simulink model "TST_InjCrv_PiIAddCor"  (R2016b)
settings: Solver=FixedStepDiscrete  StartTime=0.0  StopTime=simTime  FixedStep=sampleTime  RelTol=1e-3
values from neighbouring files (symbols this model uses):
  testCase = 1    [initTST_InjCrv_PiIAddCor_001.m]    (also in initTST_InjCrv_PiIAddCor_002.m = 2; initTST_InjCrv_PiIAddCor_003.m = 3)
libraries: simulink x7
settings Model: Creator=WF305  LastModifiedBy=WF305
settings DebuggingCC: SignalRangeChecking=error

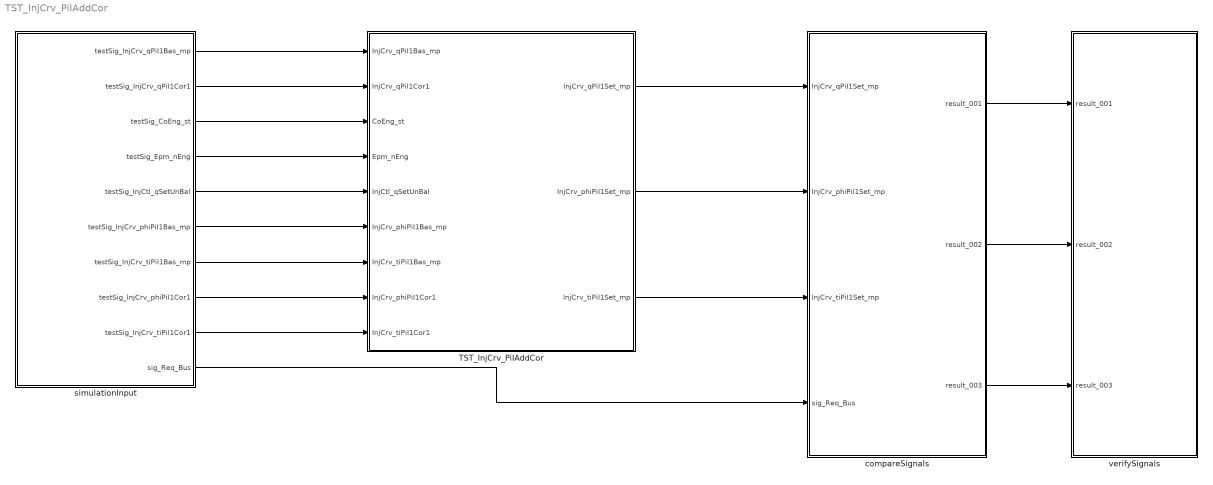
== system TST_InjCrv_PiIAddCor ==
  TST_InjCrv_PiIAddCor : Subsystem
  compareSignals : Subsystem
  simulationInput : Subsystem
  verifySignals : Subsystem
  wires:
  simulationInput/1(testSig_InjCrv_qPiI1Bas_mp) -> TST_InjCrv_PiIAddCor/1(InjCrv_qPiI1Bas_mp)
  simulationInput/2(testSig_InjCrv_qPiI1Cor1) -> TST_InjCrv_PiIAddCor/2(InjCrv_qPiI1Cor1)
  simulationInput/3(testSig_CoEng_st) -> TST_InjCrv_PiIAddCor/3(CoEng_st)
  simulationInput/4(testSig_Epm_nEng) -> TST_InjCrv_PiIAddCor/4(Epm_nEng)
  simulationInput/5(testSig_InjCtl_qSetUnBal) -> TST_InjCrv_PiIAddCor/5(InjCtl_qSetUnBal)
  simulationInput/6(testSig_InjCrv_phiPiI1Bas_mp) -> TST_InjCrv_PiIAddCor/6(InjCrv_phiPiI1Bas_mp)
  simulationInput/7(testSig_InjCrv_tiPiI1Bas_mp) -> TST_InjCrv_PiIAddCor/7(InjCrv_tiPiI1Bas_mp)
  simulationInput/8(testSig_InjCrv_phiPiI1Cor1) -> TST_InjCrv_PiIAddCor/8(InjCrv_phiPiI1Cor1)
  simulationInput/9(testSig_InjCrv_tiPiI1Cor1) -> TST_InjCrv_PiIAddCor/9(InjCrv_tiPiI1Cor1)
  TST_InjCrv_PiIAddCor/1(InjCrv_qPiI1Set_mp) -> compareSignals/1(InjCrv_qPiI1Set_mp)
  TST_InjCrv_PiIAddCor/2(InjCrv_phiPiI1Set_mp) -> compareSignals/2(InjCrv_phiPiI1Set_mp)
  TST_InjCrv_PiIAddCor/3(InjCrv_tiPiI1Set_mp) -> compareSignals/3(InjCrv_tiPiI1Set_mp)
  simulationInput/10(sig_Req_Bus) -> compareSignals/4(sig_Req_Bus)
  compareSignals/1(result_001) -> verifySignals/1(result_001)
  compareSignals/2(result_002) -> verifySignals/2(result_002)
  compareSignals/3(result_003) -> verifySignals/3(result_003)

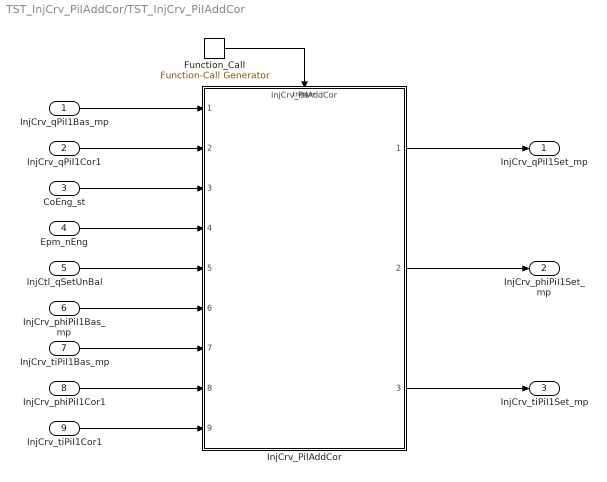
== system TST_InjCrv_PiIAddCor/TST_InjCrv_PiIAddCor ==
  InjCrv_qPiI1Bas_mp : Inport
  InjCrv_qPiI1Cor1 : Inport  Port=2
  CoEng_st : Inport  Port=3
  Epm_nEng : Inport  Port=4
  InjCtl_qSetUnBal : Inport  Port=5
  InjCrv_phiPiI1Bas_mp : Inport  Port=6
  InjCrv_tiPiI1Bas_mp : Inport  Port=7
  InjCrv_phiPiI1Cor1 : Inport  Port=8
  InjCrv_tiPiI1Cor1 : Inport  Port=9
  Function_Call : simulink/Ports & Subsystems/Function-Call Generator  sample_time=sampleTime  numberOfIterations=1
  InjCrv_PiIAddCor : ModelReference  ModelNameDialog=InjCrv_PiIAddCor  ModelReferenceVersion=1.17  TriggerPortName=function  TriggerPortTriggerType=function-call  TriggerPortStatesWhenEnabling=held
  InjCrv_qPiI1Set_mp : Outport
  InjCrv_phiPiI1Set_mp : Outport  Port=2
  InjCrv_tiPiI1Set_mp : Outport  Port=3
  wires:
  Function_Call/1 -> InjCrv_PiIAddCor/Trigger
  InjCrv_qPiI1Bas_mp/1 -> InjCrv_PiIAddCor/1
  InjCrv_qPiI1Cor1/1 -> InjCrv_PiIAddCor/2
  CoEng_st/1 -> InjCrv_PiIAddCor/3
  Epm_nEng/1 -> InjCrv_PiIAddCor/4
  InjCtl_qSetUnBal/1 -> InjCrv_PiIAddCor/5
  InjCrv_phiPiI1Bas_mp/1 -> InjCrv_PiIAddCor/6
  InjCrv_tiPiI1Bas_mp/1 -> InjCrv_PiIAddCor/7
  InjCrv_phiPiI1Cor1/1 -> InjCrv_PiIAddCor/8
  InjCrv_tiPiI1Cor1/1 -> InjCrv_PiIAddCor/9
  InjCrv_PiIAddCor/1 -> InjCrv_qPiI1Set_mp/1
  InjCrv_PiIAddCor/2 -> InjCrv_phiPiI1Set_mp/1
  InjCrv_PiIAddCor/3 -> InjCrv_tiPiI1Set_mp/1

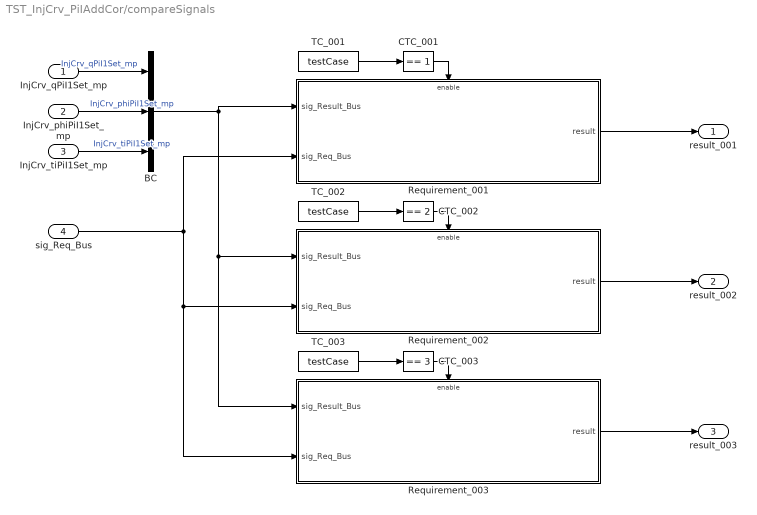
== system TST_InjCrv_PiIAddCor/compareSignals ==
  InjCrv_qPiI1Set_mp : Inport
  InjCrv_phiPiI1Set_mp : Inport  Port=2
  InjCrv_tiPiI1Set_mp : Inport  Port=3
  sig_Req_Bus : Inport  Port=4
  BC : BusCreator  Inputs=3
  CTC_001 : simulink/Logic and Bit Operations/Compare To Constant  relop===  const=1  OutDataTypeStr=boolean
  CTC_002 : simulink/Logic and Bit Operations/Compare To Constant  relop===  const=2  OutDataTypeStr=boolean
  CTC_003 : simulink/Logic and Bit Operations/Compare To Constant  relop===  const=3  OutDataTypeStr=boolean
  Requirement_001 : Subsystem
  Requirement_002 : Subsystem
  Requirement_003 : Subsystem
  TC_001 : Constant  Value=testCase
  TC_002 : Constant  Value=testCase
  TC_003 : Constant  Value=testCase
  result_001 : Outport
  result_002 : Outport  Port=2
  result_003 : Outport  Port=3
  wires:
  InjCrv_qPiI1Set_mp/1 -> BC/1  "InjCrv_qPiI1Set_mp"
  InjCrv_phiPiI1Set_mp/1 -> BC/2  "InjCrv_phiPiI1Set_mp"
  InjCrv_tiPiI1Set_mp/1 -> BC/3  "InjCrv_tiPiI1Set_mp"
  TC_001/1 -> CTC_001/1
  CTC_001/1 -> Requirement_001/Enable
  sig_Req_Bus/1 -> Requirement_002/2(sig_Req_Bus), Requirement_003/2(sig_Req_Bus), Requirement_001/2(sig_Req_Bus)
  BC/1 -> Requirement_002/1(sig_Result_Bus), Requirement_003/1(sig_Result_Bus), Requirement_001/1(sig_Result_Bus)
  Requirement_001/1(result) -> result_001/1
  TC_002/1 -> CTC_002/1
  CTC_002/1 -> Requirement_002/Enable
  Requirement_002/1(result) -> result_002/1
  TC_003/1 -> CTC_003/1
  CTC_003/1 -> Requirement_003/Enable
  Requirement_003/1(result) -> result_003/1

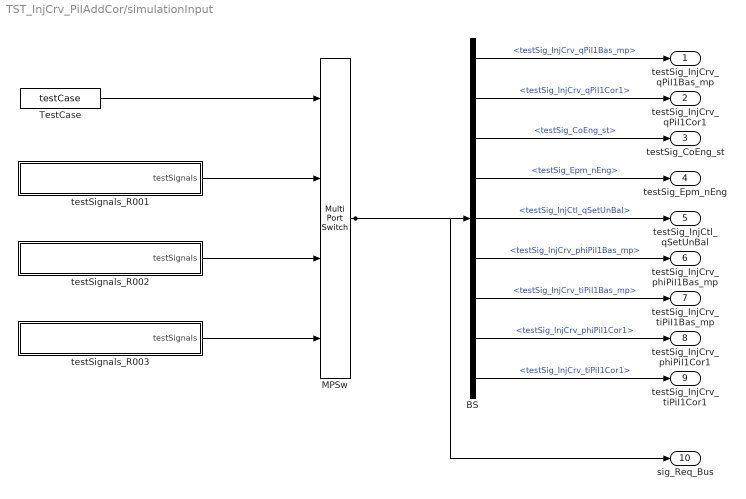
== system TST_InjCrv_PiIAddCor/simulationInput ==
  BS : BusSelector  OutputSignals=testSig_InjCrv_qPiI1Bas_mp,testSig_InjCrv_qPiI1Cor1,testSig_CoEng_st,testSig_Epm_nEng,testSig_InjCtl_qSetUnBal,testSig_InjCrv_phiPiI1Bas_mp,testSig_InjCrv_tiPiI1Bas_mp,testSig_InjCrv_phiPiI1Cor1,testSig_InjCrv_tiPiI1Cor1
  MPSw : MultiPortSwitch  SaturateOnIntegerOverflow=on  InputSameDT=on
  TestCase : Constant  Value=testCase
  testSignals_R001 : Subsystem
  testSignals_R002 : Subsystem
  testSignals_R003 : Subsystem
  testSig_InjCrv_qPiI1Bas_mp : Outport
  testSig_InjCrv_qPiI1Cor1 : Outport  Port=2
  testSig_CoEng_st : Outport  Port=3
  testSig_Epm_nEng : Outport  Port=4
  testSig_InjCtl_qSetUnBal : Outport  Port=5
  testSig_InjCrv_phiPiI1Bas_mp : Outport  Port=6
  testSig_InjCrv_tiPiI1Bas_mp : Outport  Port=7
  testSig_InjCrv_phiPiI1Cor1 : Outport  Port=8
  testSig_InjCrv_tiPiI1Cor1 : Outport  Port=9
  sig_Req_Bus : Outport  Port=10
  wires:
  BS/1 -> testSig_InjCrv_qPiI1Bas_mp/1  "<testSig_InjCrv_qPiI1Bas_mp>"
  BS/2 -> testSig_InjCrv_qPiI1Cor1/1  "<testSig_InjCrv_qPiI1Cor1>"
  BS/3 -> testSig_CoEng_st/1  "<testSig_CoEng_st>"
  BS/4 -> testSig_Epm_nEng/1  "<testSig_Epm_nEng>"
  BS/5 -> testSig_InjCtl_qSetUnBal/1  "<testSig_InjCtl_qSetUnBal>"
  BS/6 -> testSig_InjCrv_phiPiI1Bas_mp/1  "<testSig_InjCrv_phiPiI1Bas_mp>"
  BS/7 -> testSig_InjCrv_tiPiI1Bas_mp/1  "<testSig_InjCrv_tiPiI1Bas_mp>"
  BS/8 -> testSig_InjCrv_phiPiI1Cor1/1  "<testSig_InjCrv_phiPiI1Cor1>"
  BS/9 -> testSig_InjCrv_tiPiI1Cor1/1  "<testSig_InjCrv_tiPiI1Cor1>"
  MPSw/1 -> BS/1, sig_Req_Bus/1
  TestCase/1 -> MPSw/1
  testSignals_R001/1(testSignals) -> MPSw/2
  testSignals_R002/1(testSignals) -> MPSw/3
  testSignals_R003/1(testSignals) -> MPSw/4

== system TST_InjCrv_PiIAddCor/verifySignals ==
  result_001 : Inport
  result_002 : Inport  Port=2
  result_003 : Inport  Port=3
  Assertion_001 : Assertion  Enabled=off
  Assertion_002 : Assertion  Enabled=off
  Assertion_003 : Assertion  Enabled=off
  wires:
  result_001/1 -> Assertion_001/1
  result_002/1 -> Assertion_002/1
  result_003/1 -> Assertion_003/1

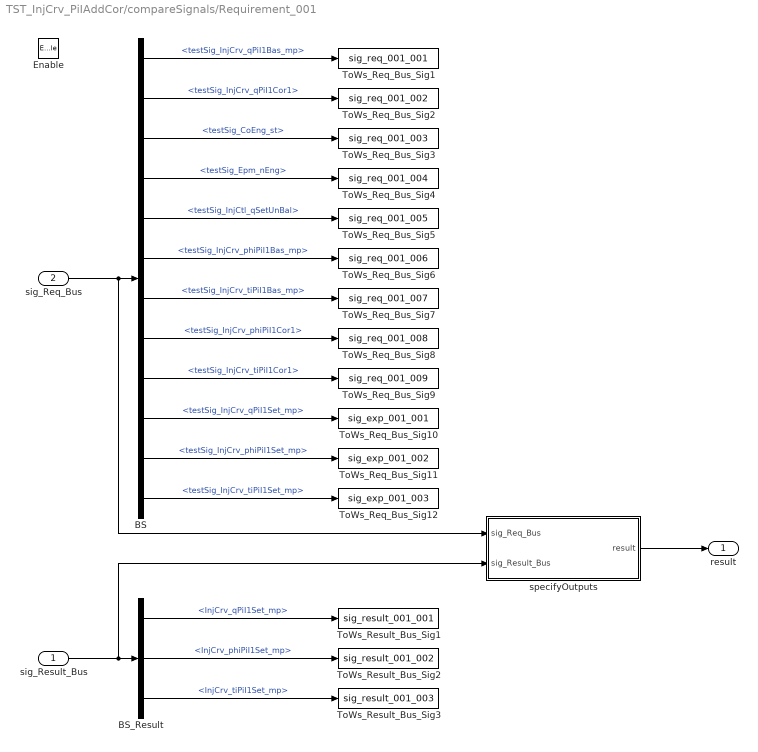
== system TST_InjCrv_PiIAddCor/compareSignals/Requirement_001 ==
  sig_Result_Bus : Inport
  sig_Req_Bus : Inport  Port=2
  Enable : EnablePort
  BS : BusSelector  OutputSignals=testSig_InjCrv_qPiI1Bas_mp,testSig_InjCrv_qPiI1Cor1,testSig_CoEng_st,testSig_Epm_nEng,testSig_InjCtl_qSetUnBal,testSig_InjCrv_phiPiI1Bas_mp,testSig_InjCrv_tiPiI1Bas_mp,testSig_InjCrv_phiPiI1Cor1,testSig_InjCrv_tiPiI1Cor1,testSig_InjCrv_qPiI1Set_mp,testSig_InjCrv_phiPiI1Set_mp,testSig_InjCrv_tiPiI1Set_mp
  BS_Result : BusSelector  OutputSignals=InjCrv_qPiI1Set_mp,InjCrv_phiPiI1Set_mp,InjCrv_tiPiI1Set_mp
  ToWs_Req_Bus_Sig1 : ToWorkspace  VariableName=sig_req_001_001  SaveFormat=Structure With Time
  ToWs_Req_Bus_Sig10 : ToWorkspace  VariableName=sig_exp_001_001  SaveFormat=Structure With Time
  ToWs_Req_Bus_Sig11 : ToWorkspace  VariableName=sig_exp_001_002  SaveFormat=Structure With Time
  ToWs_Req_Bus_Sig12 : ToWorkspace  VariableName=sig_exp_001_003  SaveFormat=Structure With Time
  ToWs_Req_Bus_Sig2 : ToWorkspace  VariableName=sig_req_001_002  SaveFormat=Structure With Time
  ToWs_Req_Bus_Sig3 : ToWorkspace  VariableName=sig_req_001_003  SaveFormat=Structure With Time
  ToWs_Req_Bus_Sig4 : ToWorkspace  VariableName=sig_req_001_004  SaveFormat=Structure With Time
  ToWs_Req_Bus_Sig5 : ToWorkspace  VariableName=sig_req_001_005  SaveFormat=Structure With Time
  ToWs_Req_Bus_Sig6 : ToWorkspace  VariableName=sig_req_001_006  SaveFormat=Structure With Time
  ToWs_Req_Bus_Sig7 : ToWorkspace  VariableName=sig_req_001_007  SaveFormat=Structure With Time
  ToWs_Req_Bus_Sig8 : ToWorkspace  VariableName=sig_req_001_008  SaveFormat=Structure With Time
  ToWs_Req_Bus_Sig9 : ToWorkspace  VariableName=sig_req_001_009  SaveFormat=Structure With Time
  ToWs_Result_Bus_Sig1 : ToWorkspace  VariableName=sig_result_001_001  SaveFormat=Structure With Time
  ToWs_Result_Bus_Sig2 : ToWorkspace  VariableName=sig_result_001_002  SaveFormat=Structure With Time
  ToWs_Result_Bus_Sig3 : ToWorkspace  VariableName=sig_result_001_003  SaveFormat=Structure With Time
  specifyOutputs : Subsystem
  result : Outport
  wires:
  sig_Req_Bus/1 -> BS/1, specifyOutputs/1(sig_Req_Bus)
  BS/1 -> ToWs_Req_Bus_Sig1/1  "<testSig_InjCrv_qPiI1Bas_mp>"
  BS/2 -> ToWs_Req_Bus_Sig2/1  "<testSig_InjCrv_qPiI1Cor1>"
  BS/3 -> ToWs_Req_Bus_Sig3/1  "<testSig_CoEng_st>"
  BS/4 -> ToWs_Req_Bus_Sig4/1  "<testSig_Epm_nEng>"
  BS/5 -> ToWs_Req_Bus_Sig5/1  "<testSig_InjCtl_qSetUnBal>"
  BS/6 -> ToWs_Req_Bus_Sig6/1  "<testSig_InjCrv_phiPiI1Bas_mp>"
  BS/7 -> ToWs_Req_Bus_Sig7/1  "<testSig_InjCrv_tiPiI1Bas_mp>"
  BS/8 -> ToWs_Req_Bus_Sig8/1  "<testSig_InjCrv_phiPiI1Cor1>"
  BS/9 -> ToWs_Req_Bus_Sig9/1  "<testSig_InjCrv_tiPiI1Cor1>"
  BS/10 -> ToWs_Req_Bus_Sig10/1  "<testSig_InjCrv_qPiI1Set_mp>"
  BS/11 -> ToWs_Req_Bus_Sig11/1  "<testSig_InjCrv_phiPiI1Set_mp>"
  BS/12 -> ToWs_Req_Bus_Sig12/1  "<testSig_InjCrv_tiPiI1Set_mp>"
  sig_Result_Bus/1 -> BS_Result/1, specifyOutputs/2(sig_Result_Bus)
  BS_Result/1 -> ToWs_Result_Bus_Sig1/1  "<InjCrv_qPiI1Set_mp>"
  BS_Result/2 -> ToWs_Result_Bus_Sig2/1  "<InjCrv_phiPiI1Set_mp>"
  BS_Result/3 -> ToWs_Result_Bus_Sig3/1  "<InjCrv_tiPiI1Set_mp>"
  specifyOutputs/1(result) -> result/1

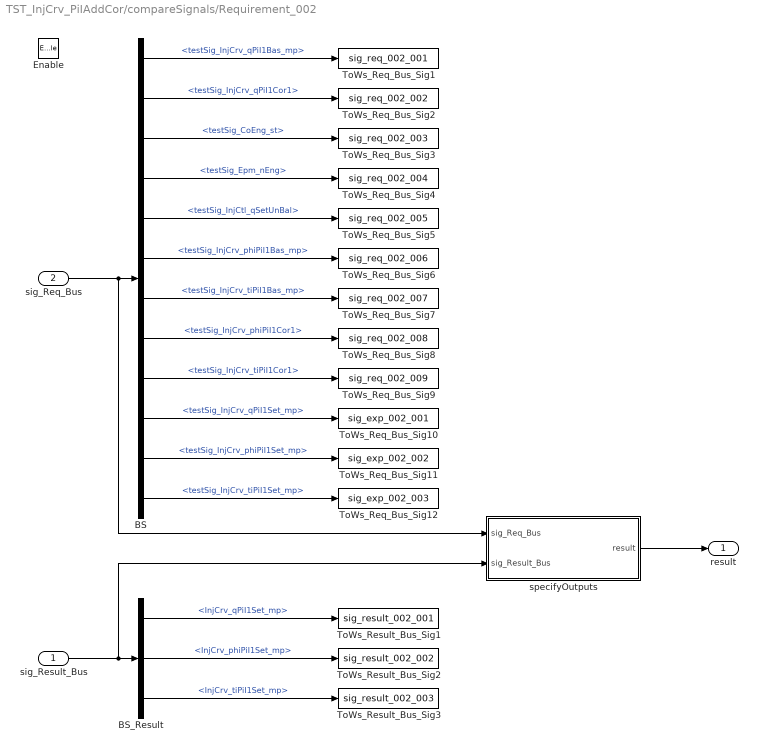
== system TST_InjCrv_PiIAddCor/compareSignals/Requirement_002 ==
  sig_Result_Bus : Inport
  sig_Req_Bus : Inport  Port=2
  Enable : EnablePort
  BS : BusSelector  OutputSignals=testSig_InjCrv_qPiI1Bas_mp,testSig_InjCrv_qPiI1Cor1,testSig_CoEng_st,testSig_Epm_nEng,testSig_InjCtl_qSetUnBal,testSig_InjCrv_phiPiI1Bas_mp,testSig_InjCrv_tiPiI1Bas_mp,testSig_InjCrv_phiPiI1Cor1,testSig_InjCrv_tiPiI1Cor1,testSig_InjCrv_qPiI1Set_mp,testSig_InjCrv_phiPiI1Set_mp,testSig_InjCrv_tiPiI1Set_mp
  BS_Result : BusSelector  OutputSignals=InjCrv_qPiI1Set_mp,InjCrv_phiPiI1Set_mp,InjCrv_tiPiI1Set_mp
  ToWs_Req_Bus_Sig1 : ToWorkspace  VariableName=sig_req_002_001  SaveFormat=Structure With Time
  ToWs_Req_Bus_Sig10 : ToWorkspace  VariableName=sig_exp_002_001  SaveFormat=Structure With Time
  ToWs_Req_Bus_Sig11 : ToWorkspace  VariableName=sig_exp_002_002  SaveFormat=Structure With Time
  ToWs_Req_Bus_Sig12 : ToWorkspace  VariableName=sig_exp_002_003  SaveFormat=Structure With Time
  ToWs_Req_Bus_Sig2 : ToWorkspace  VariableName=sig_req_002_002  SaveFormat=Structure With Time
  ToWs_Req_Bus_Sig3 : ToWorkspace  VariableName=sig_req_002_003  SaveFormat=Structure With Time
  ToWs_Req_Bus_Sig4 : ToWorkspace  VariableName=sig_req_002_004  SaveFormat=Structure With Time
  ToWs_Req_Bus_Sig5 : ToWorkspace  VariableName=sig_req_002_005  SaveFormat=Structure With Time
  ToWs_Req_Bus_Sig6 : ToWorkspace  VariableName=sig_req_002_006  SaveFormat=Structure With Time
  ToWs_Req_Bus_Sig7 : ToWorkspace  VariableName=sig_req_002_007  SaveFormat=Structure With Time
  ToWs_Req_Bus_Sig8 : ToWorkspace  VariableName=sig_req_002_008  SaveFormat=Structure With Time
  ToWs_Req_Bus_Sig9 : ToWorkspace  VariableName=sig_req_002_009  SaveFormat=Structure With Time
  ToWs_Result_Bus_Sig1 : ToWorkspace  VariableName=sig_result_002_001  SaveFormat=Structure With Time
  ToWs_Result_Bus_Sig2 : ToWorkspace  VariableName=sig_result_002_002  SaveFormat=Structure With Time
  ToWs_Result_Bus_Sig3 : ToWorkspace  VariableName=sig_result_002_003  SaveFormat=Structure With Time
  specifyOutputs : Subsystem
  result : Outport
  wires:
  sig_Req_Bus/1 -> BS/1, specifyOutputs/1(sig_Req_Bus)
  BS/1 -> ToWs_Req_Bus_Sig1/1  "<testSig_InjCrv_qPiI1Bas_mp>"
  BS/2 -> ToWs_Req_Bus_Sig2/1  "<testSig_InjCrv_qPiI1Cor1>"
  BS/3 -> ToWs_Req_Bus_Sig3/1  "<testSig_CoEng_st>"
  BS/4 -> ToWs_Req_Bus_Sig4/1  "<testSig_Epm_nEng>"
  BS/5 -> ToWs_Req_Bus_Sig5/1  "<testSig_InjCtl_qSetUnBal>"
  BS/6 -> ToWs_Req_Bus_Sig6/1  "<testSig_InjCrv_phiPiI1Bas_mp>"
  BS/7 -> ToWs_Req_Bus_Sig7/1  "<testSig_InjCrv_tiPiI1Bas_mp>"
  BS/8 -> ToWs_Req_Bus_Sig8/1  "<testSig_InjCrv_phiPiI1Cor1>"
  BS/9 -> ToWs_Req_Bus_Sig9/1  "<testSig_InjCrv_tiPiI1Cor1>"
  BS/10 -> ToWs_Req_Bus_Sig10/1  "<testSig_InjCrv_qPiI1Set_mp>"
  BS/11 -> ToWs_Req_Bus_Sig11/1  "<testSig_InjCrv_phiPiI1Set_mp>"
  BS/12 -> ToWs_Req_Bus_Sig12/1  "<testSig_InjCrv_tiPiI1Set_mp>"
  sig_Result_Bus/1 -> BS_Result/1, specifyOutputs/2(sig_Result_Bus)
  BS_Result/1 -> ToWs_Result_Bus_Sig1/1  "<InjCrv_qPiI1Set_mp>"
  BS_Result/2 -> ToWs_Result_Bus_Sig2/1  "<InjCrv_phiPiI1Set_mp>"
  BS_Result/3 -> ToWs_Result_Bus_Sig3/1  "<InjCrv_tiPiI1Set_mp>"
  specifyOutputs/1(result) -> result/1

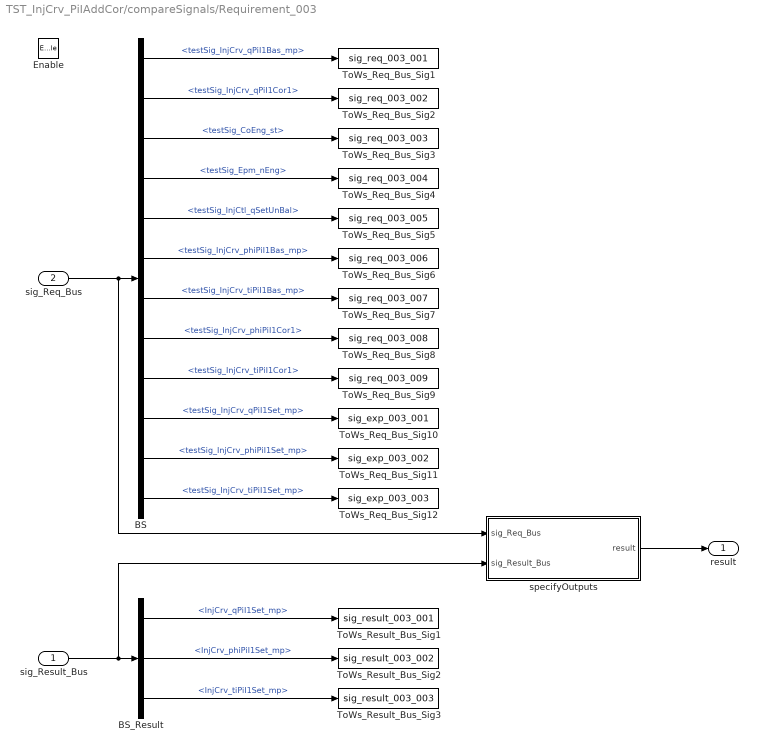
== system TST_InjCrv_PiIAddCor/compareSignals/Requirement_003 ==
  sig_Result_Bus : Inport
  sig_Req_Bus : Inport  Port=2
  Enable : EnablePort
  BS : BusSelector  OutputSignals=testSig_InjCrv_qPiI1Bas_mp,testSig_InjCrv_qPiI1Cor1,testSig_CoEng_st,testSig_Epm_nEng,testSig_InjCtl_qSetUnBal,testSig_InjCrv_phiPiI1Bas_mp,testSig_InjCrv_tiPiI1Bas_mp,testSig_InjCrv_phiPiI1Cor1,testSig_InjCrv_tiPiI1Cor1,testSig_InjCrv_qPiI1Set_mp,testSig_InjCrv_phiPiI1Set_mp,testSig_InjCrv_tiPiI1Set_mp
  BS_Result : BusSelector  OutputSignals=InjCrv_qPiI1Set_mp,InjCrv_phiPiI1Set_mp,InjCrv_tiPiI1Set_mp
  ToWs_Req_Bus_Sig1 : ToWorkspace  VariableName=sig_req_003_001  SaveFormat=Structure With Time
  ToWs_Req_Bus_Sig10 : ToWorkspace  VariableName=sig_exp_003_001  SaveFormat=Structure With Time
  ToWs_Req_Bus_Sig11 : ToWorkspace  VariableName=sig_exp_003_002  SaveFormat=Structure With Time
  ToWs_Req_Bus_Sig12 : ToWorkspace  VariableName=sig_exp_003_003  SaveFormat=Structure With Time
  ToWs_Req_Bus_Sig2 : ToWorkspace  VariableName=sig_req_003_002  SaveFormat=Structure With Time
  ToWs_Req_Bus_Sig3 : ToWorkspace  VariableName=sig_req_003_003  SaveFormat=Structure With Time
  ToWs_Req_Bus_Sig4 : ToWorkspace  VariableName=sig_req_003_004  SaveFormat=Structure With Time
  ToWs_Req_Bus_Sig5 : ToWorkspace  VariableName=sig_req_003_005  SaveFormat=Structure With Time
  ToWs_Req_Bus_Sig6 : ToWorkspace  VariableName=sig_req_003_006  SaveFormat=Structure With Time
  ToWs_Req_Bus_Sig7 : ToWorkspace  VariableName=sig_req_003_007  SaveFormat=Structure With Time
  ToWs_Req_Bus_Sig8 : ToWorkspace  VariableName=sig_req_003_008  SaveFormat=Structure With Time
  ToWs_Req_Bus_Sig9 : ToWorkspace  VariableName=sig_req_003_009  SaveFormat=Structure With Time
  ToWs_Result_Bus_Sig1 : ToWorkspace  VariableName=sig_result_003_001  SaveFormat=Structure With Time
  ToWs_Result_Bus_Sig2 : ToWorkspace  VariableName=sig_result_003_002  SaveFormat=Structure With Time
  ToWs_Result_Bus_Sig3 : ToWorkspace  VariableName=sig_result_003_003  SaveFormat=Structure With Time
  specifyOutputs : Subsystem
  result : Outport
  wires:
  sig_Req_Bus/1 -> BS/1, specifyOutputs/1(sig_Req_Bus)
  BS/1 -> ToWs_Req_Bus_Sig1/1  "<testSig_InjCrv_qPiI1Bas_mp>"
  BS/2 -> ToWs_Req_Bus_Sig2/1  "<testSig_InjCrv_qPiI1Cor1>"
  BS/3 -> ToWs_Req_Bus_Sig3/1  "<testSig_CoEng_st>"
  BS/4 -> ToWs_Req_Bus_Sig4/1  "<testSig_Epm_nEng>"
  BS/5 -> ToWs_Req_Bus_Sig5/1  "<testSig_InjCtl_qSetUnBal>"
  BS/6 -> ToWs_Req_Bus_Sig6/1  "<testSig_InjCrv_phiPiI1Bas_mp>"
  BS/7 -> ToWs_Req_Bus_Sig7/1  "<testSig_InjCrv_tiPiI1Bas_mp>"
  BS/8 -> ToWs_Req_Bus_Sig8/1  "<testSig_InjCrv_phiPiI1Cor1>"
  BS/9 -> ToWs_Req_Bus_Sig9/1  "<testSig_InjCrv_tiPiI1Cor1>"
  BS/10 -> ToWs_Req_Bus_Sig10/1  "<testSig_InjCrv_qPiI1Set_mp>"
  BS/11 -> ToWs_Req_Bus_Sig11/1  "<testSig_InjCrv_phiPiI1Set_mp>"
  BS/12 -> ToWs_Req_Bus_Sig12/1  "<testSig_InjCrv_tiPiI1Set_mp>"
  sig_Result_Bus/1 -> BS_Result/1, specifyOutputs/2(sig_Result_Bus)
  BS_Result/1 -> ToWs_Result_Bus_Sig1/1  "<InjCrv_qPiI1Set_mp>"
  BS_Result/2 -> ToWs_Result_Bus_Sig2/1  "<InjCrv_phiPiI1Set_mp>"
  BS_Result/3 -> ToWs_Result_Bus_Sig3/1  "<InjCrv_tiPiI1Set_mp>"
  specifyOutputs/1(result) -> result/1

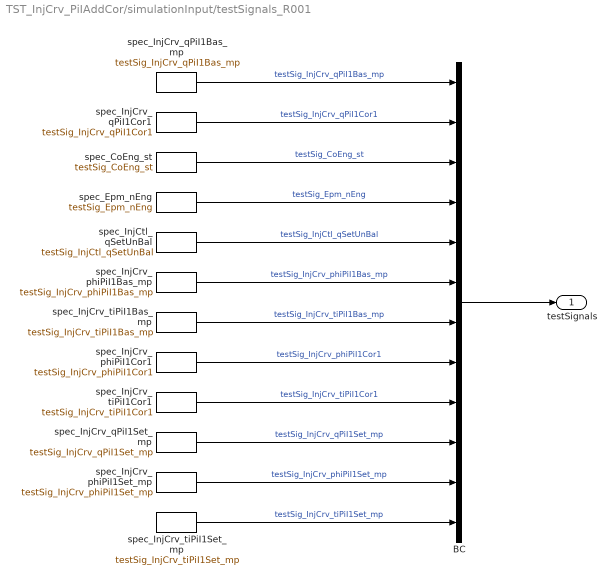
== system TST_InjCrv_PiIAddCor/simulationInput/testSignals_R001 ==
  BC : BusCreator  Inputs=12
  spec_CoEng_st : FromWorkspace  VariableName=testSig_CoEng_st  Interpolate=off  OutputAfterFinalValue=Holding final value
  spec_Epm_nEng : FromWorkspace  VariableName=testSig_Epm_nEng  Interpolate=off  OutputAfterFinalValue=Holding final value
  spec_InjCrv_phiPiI1Bas_mp : FromWorkspace  VariableName=testSig_InjCrv_phiPiI1Bas_mp  Interpolate=off  OutputAfterFinalValue=Holding final value
  spec_InjCrv_phiPiI1Cor1 : FromWorkspace  VariableName=testSig_InjCrv_phiPiI1Cor1  Interpolate=off  OutputAfterFinalValue=Holding final value
  spec_InjCrv_phiPiI1Set_mp : FromWorkspace  VariableName=testSig_InjCrv_phiPiI1Set_mp  Interpolate=off  OutputAfterFinalValue=Holding final value
  spec_InjCrv_qPiI1Bas_mp : FromWorkspace  VariableName=testSig_InjCrv_qPiI1Bas_mp  Interpolate=off  OutputAfterFinalValue=Holding final value
  spec_InjCrv_qPiI1Cor1 : FromWorkspace  VariableName=testSig_InjCrv_qPiI1Cor1  Interpolate=off  OutputAfterFinalValue=Holding final value
  spec_InjCrv_qPiI1Set_mp : FromWorkspace  VariableName=testSig_InjCrv_qPiI1Set_mp  Interpolate=off  OutputAfterFinalValue=Holding final value
  spec_InjCrv_tiPiI1Bas_mp : FromWorkspace  VariableName=testSig_InjCrv_tiPiI1Bas_mp  Interpolate=off  OutputAfterFinalValue=Holding final value
  spec_InjCrv_tiPiI1Cor1 : FromWorkspace  VariableName=testSig_InjCrv_tiPiI1Cor1  Interpolate=off  OutputAfterFinalValue=Holding final value
  spec_InjCrv_tiPiI1Set_mp : FromWorkspace  VariableName=testSig_InjCrv_tiPiI1Set_mp  Interpolate=off  OutputAfterFinalValue=Holding final value
  spec_InjCtl_qSetUnBal : FromWorkspace  VariableName=testSig_InjCtl_qSetUnBal  Interpolate=off  OutputAfterFinalValue=Holding final value
  testSignals : Outport
  wires:
  BC/1 -> testSignals/1
  spec_InjCrv_qPiI1Bas_mp/1 -> BC/1  "testSig_InjCrv_qPiI1Bas_mp"
  spec_InjCrv_qPiI1Cor1/1 -> BC/2  "testSig_InjCrv_qPiI1Cor1"
  spec_CoEng_st/1 -> BC/3  "testSig_CoEng_st"
  spec_Epm_nEng/1 -> BC/4  "testSig_Epm_nEng"
  spec_InjCtl_qSetUnBal/1 -> BC/5  "testSig_InjCtl_qSetUnBal"
  spec_InjCrv_phiPiI1Bas_mp/1 -> BC/6  "testSig_InjCrv_phiPiI1Bas_mp"
  spec_InjCrv_tiPiI1Bas_mp/1 -> BC/7  "testSig_InjCrv_tiPiI1Bas_mp"
  spec_InjCrv_phiPiI1Cor1/1 -> BC/8  "testSig_InjCrv_phiPiI1Cor1"
  spec_InjCrv_tiPiI1Cor1/1 -> BC/9  "testSig_InjCrv_tiPiI1Cor1"
  spec_InjCrv_qPiI1Set_mp/1 -> BC/10  "testSig_InjCrv_qPiI1Set_mp"
  spec_InjCrv_phiPiI1Set_mp/1 -> BC/11  "testSig_InjCrv_phiPiI1Set_mp"
  spec_InjCrv_tiPiI1Set_mp/1 -> BC/12  "testSig_InjCrv_tiPiI1Set_mp"

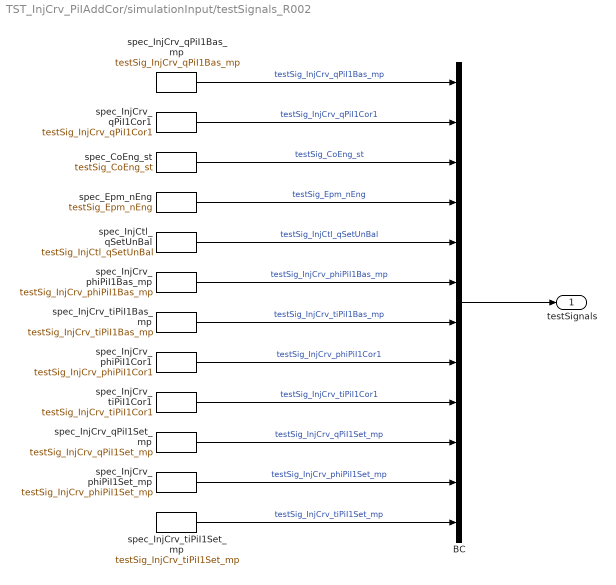
== system TST_InjCrv_PiIAddCor/simulationInput/testSignals_R002 ==
  BC : BusCreator  Inputs=12
  spec_CoEng_st : FromWorkspace  VariableName=testSig_CoEng_st  Interpolate=off  OutputAfterFinalValue=Holding final value
  spec_Epm_nEng : FromWorkspace  VariableName=testSig_Epm_nEng  Interpolate=off  OutputAfterFinalValue=Holding final value
  spec_InjCrv_phiPiI1Bas_mp : FromWorkspace  VariableName=testSig_InjCrv_phiPiI1Bas_mp  Interpolate=off  OutputAfterFinalValue=Holding final value
  spec_InjCrv_phiPiI1Cor1 : FromWorkspace  VariableName=testSig_InjCrv_phiPiI1Cor1  Interpolate=off  OutputAfterFinalValue=Holding final value
  spec_InjCrv_phiPiI1Set_mp : FromWorkspace  VariableName=testSig_InjCrv_phiPiI1Set_mp  Interpolate=off  OutputAfterFinalValue=Holding final value
  spec_InjCrv_qPiI1Bas_mp : FromWorkspace  VariableName=testSig_InjCrv_qPiI1Bas_mp  Interpolate=off  OutputAfterFinalValue=Holding final value
  spec_InjCrv_qPiI1Cor1 : FromWorkspace  VariableName=testSig_InjCrv_qPiI1Cor1  Interpolate=off  OutputAfterFinalValue=Holding final value
  spec_InjCrv_qPiI1Set_mp : FromWorkspace  VariableName=testSig_InjCrv_qPiI1Set_mp  Interpolate=off  OutputAfterFinalValue=Holding final value
  spec_InjCrv_tiPiI1Bas_mp : FromWorkspace  VariableName=testSig_InjCrv_tiPiI1Bas_mp  Interpolate=off  OutputAfterFinalValue=Holding final value
  spec_InjCrv_tiPiI1Cor1 : FromWorkspace  VariableName=testSig_InjCrv_tiPiI1Cor1  Interpolate=off  OutputAfterFinalValue=Holding final value
  spec_InjCrv_tiPiI1Set_mp : FromWorkspace  VariableName=testSig_InjCrv_tiPiI1Set_mp  Interpolate=off  OutputAfterFinalValue=Holding final value
  spec_InjCtl_qSetUnBal : FromWorkspace  VariableName=testSig_InjCtl_qSetUnBal  Interpolate=off  OutputAfterFinalValue=Holding final value
  testSignals : Outport
  wires:
  BC/1 -> testSignals/1
  spec_InjCrv_qPiI1Bas_mp/1 -> BC/1  "testSig_InjCrv_qPiI1Bas_mp"
  spec_InjCrv_qPiI1Cor1/1 -> BC/2  "testSig_InjCrv_qPiI1Cor1"
  spec_CoEng_st/1 -> BC/3  "testSig_CoEng_st"
  spec_Epm_nEng/1 -> BC/4  "testSig_Epm_nEng"
  spec_InjCtl_qSetUnBal/1 -> BC/5  "testSig_InjCtl_qSetUnBal"
  spec_InjCrv_phiPiI1Bas_mp/1 -> BC/6  "testSig_InjCrv_phiPiI1Bas_mp"
  spec_InjCrv_tiPiI1Bas_mp/1 -> BC/7  "testSig_InjCrv_tiPiI1Bas_mp"
  spec_InjCrv_phiPiI1Cor1/1 -> BC/8  "testSig_InjCrv_phiPiI1Cor1"
  spec_InjCrv_tiPiI1Cor1/1 -> BC/9  "testSig_InjCrv_tiPiI1Cor1"
  spec_InjCrv_qPiI1Set_mp/1 -> BC/10  "testSig_InjCrv_qPiI1Set_mp"
  spec_InjCrv_phiPiI1Set_mp/1 -> BC/11  "testSig_InjCrv_phiPiI1Set_mp"
  spec_InjCrv_tiPiI1Set_mp/1 -> BC/12  "testSig_InjCrv_tiPiI1Set_mp"

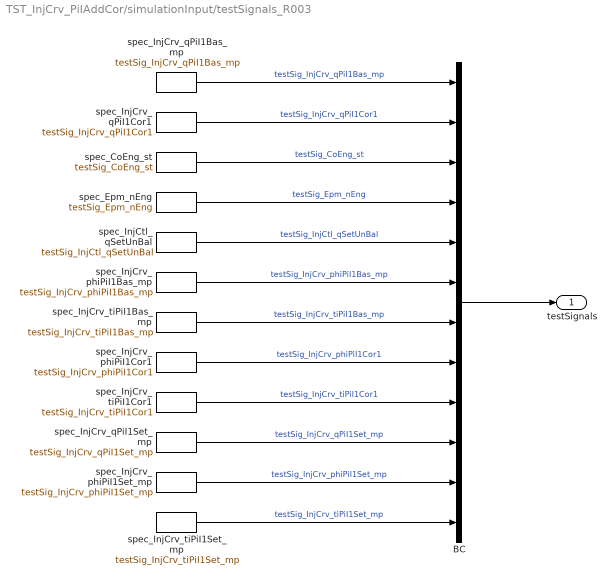
== system TST_InjCrv_PiIAddCor/simulationInput/testSignals_R003 ==
  BC : BusCreator  Inputs=12
  spec_CoEng_st : FromWorkspace  VariableName=testSig_CoEng_st  Interpolate=off  OutputAfterFinalValue=Holding final value
  spec_Epm_nEng : FromWorkspace  VariableName=testSig_Epm_nEng  Interpolate=off  OutputAfterFinalValue=Holding final value
  spec_InjCrv_phiPiI1Bas_mp : FromWorkspace  VariableName=testSig_InjCrv_phiPiI1Bas_mp  Interpolate=off  OutputAfterFinalValue=Holding final value
  spec_InjCrv_phiPiI1Cor1 : FromWorkspace  VariableName=testSig_InjCrv_phiPiI1Cor1  Interpolate=off  OutputAfterFinalValue=Holding final value
  spec_InjCrv_phiPiI1Set_mp : FromWorkspace  VariableName=testSig_InjCrv_phiPiI1Set_mp  Interpolate=off  OutputAfterFinalValue=Holding final value
  spec_InjCrv_qPiI1Bas_mp : FromWorkspace  VariableName=testSig_InjCrv_qPiI1Bas_mp  Interpolate=off  OutputAfterFinalValue=Holding final value
  spec_InjCrv_qPiI1Cor1 : FromWorkspace  VariableName=testSig_InjCrv_qPiI1Cor1  Interpolate=off  OutputAfterFinalValue=Holding final value
  spec_InjCrv_qPiI1Set_mp : FromWorkspace  VariableName=testSig_InjCrv_qPiI1Set_mp  Interpolate=off  OutputAfterFinalValue=Holding final value
  spec_InjCrv_tiPiI1Bas_mp : FromWorkspace  VariableName=testSig_InjCrv_tiPiI1Bas_mp  Interpolate=off  OutputAfterFinalValue=Holding final value
  spec_InjCrv_tiPiI1Cor1 : FromWorkspace  VariableName=testSig_InjCrv_tiPiI1Cor1  Interpolate=off  OutputAfterFinalValue=Holding final value
  spec_InjCrv_tiPiI1Set_mp : FromWorkspace  VariableName=testSig_InjCrv_tiPiI1Set_mp  Interpolate=off  OutputAfterFinalValue=Holding final value
  spec_InjCtl_qSetUnBal : FromWorkspace  VariableName=testSig_InjCtl_qSetUnBal  Interpolate=off  OutputAfterFinalValue=Holding final value
  testSignals : Outport
  wires:
  BC/1 -> testSignals/1
  spec_InjCrv_qPiI1Bas_mp/1 -> BC/1  "testSig_InjCrv_qPiI1Bas_mp"
  spec_InjCrv_qPiI1Cor1/1 -> BC/2  "testSig_InjCrv_qPiI1Cor1"
  spec_CoEng_st/1 -> BC/3  "testSig_CoEng_st"
  spec_Epm_nEng/1 -> BC/4  "testSig_Epm_nEng"
  spec_InjCtl_qSetUnBal/1 -> BC/5  "testSig_InjCtl_qSetUnBal"
  spec_InjCrv_phiPiI1Bas_mp/1 -> BC/6  "testSig_InjCrv_phiPiI1Bas_mp"
  spec_InjCrv_tiPiI1Bas_mp/1 -> BC/7  "testSig_InjCrv_tiPiI1Bas_mp"
  spec_InjCrv_phiPiI1Cor1/1 -> BC/8  "testSig_InjCrv_phiPiI1Cor1"
  spec_InjCrv_tiPiI1Cor1/1 -> BC/9  "testSig_InjCrv_tiPiI1Cor1"
  spec_InjCrv_qPiI1Set_mp/1 -> BC/10  "testSig_InjCrv_qPiI1Set_mp"
  spec_InjCrv_phiPiI1Set_mp/1 -> BC/11  "testSig_InjCrv_phiPiI1Set_mp"
  spec_InjCrv_tiPiI1Set_mp/1 -> BC/12  "testSig_InjCrv_tiPiI1Set_mp"

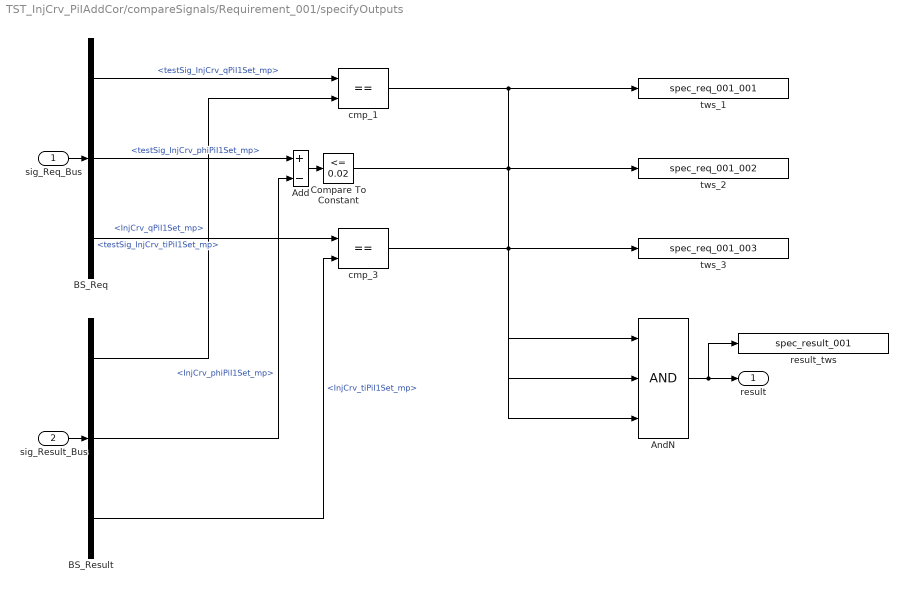
== system TST_InjCrv_PiIAddCor/compareSignals/Requirement_001/specifyOutputs ==
  sig_Req_Bus : Inport
  sig_Result_Bus : Inport  Port=2
  Add : Sum  Inputs=+-
  AndN : Logic  Inputs=3
  BS_Req : BusSelector  OutputSignals=testSig_InjCrv_qPiI1Set_mp,testSig_InjCrv_phiPiI1Set_mp,testSig_InjCrv_tiPiI1Set_mp
  BS_Result : BusSelector  OutputSignals=InjCrv_qPiI1Set_mp,InjCrv_phiPiI1Set_mp,InjCrv_tiPiI1Set_mp
  Compare To Constant : simulink/Logic and Bit Operations/Compare To Constant  relop=<=  const=0.02  OutDataTypeStr=boolean
  cmp_1 : RelationalOperator  Operator===  RndMeth=Nearest  InputSameDT=on
  cmp_3 : RelationalOperator  Operator===  RndMeth=Nearest  InputSameDT=on
  result_tws : ToWorkspace  VariableName=spec_result_001
  tws_1 : ToWorkspace  VariableName=spec_req_001_001
  tws_2 : ToWorkspace  VariableName=spec_req_001_002
  tws_3 : ToWorkspace  VariableName=spec_req_001_003
  result : Outport
  wires:
  sig_Req_Bus/1 -> BS_Req/1
  sig_Result_Bus/1 -> BS_Result/1
  AndN/1 -> result/1, result_tws/1
  BS_Req/1 -> cmp_1/1  "<testSig_InjCrv_qPiI1Set_mp>"
  BS_Result/1 -> cmp_1/2  "<InjCrv_qPiI1Set_mp>"
  cmp_1/1 -> tws_1/1, AndN/1
  BS_Req/2 -> Add/1  "<testSig_InjCrv_phiPiI1Set_mp>"
  BS_Result/2 -> Add/2  "<InjCrv_phiPiI1Set_mp>"
  Compare To Constant/1 -> tws_2/1, AndN/2
  BS_Req/3 -> cmp_3/1  "<testSig_InjCrv_tiPiI1Set_mp>"
  BS_Result/3 -> cmp_3/2  "<InjCrv_tiPiI1Set_mp>"
  cmp_3/1 -> tws_3/1, AndN/3
  Add/1 -> Compare To Constant/1

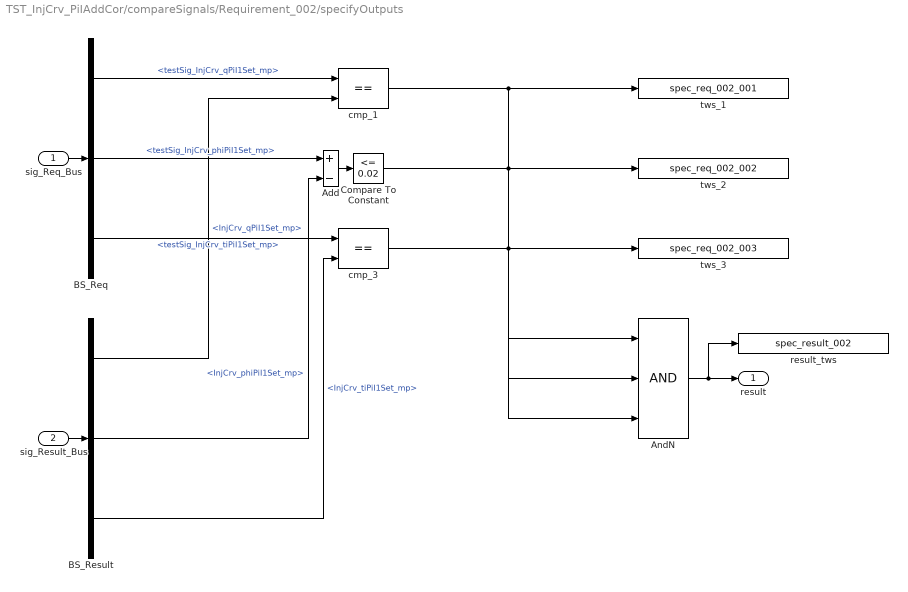
== system TST_InjCrv_PiIAddCor/compareSignals/Requirement_002/specifyOutputs ==
  sig_Req_Bus : Inport
  sig_Result_Bus : Inport  Port=2
  Add : Sum  Inputs=+-
  AndN : Logic  Inputs=3
  BS_Req : BusSelector  OutputSignals=testSig_InjCrv_qPiI1Set_mp,testSig_InjCrv_phiPiI1Set_mp,testSig_InjCrv_tiPiI1Set_mp
  BS_Result : BusSelector  OutputSignals=InjCrv_qPiI1Set_mp,InjCrv_phiPiI1Set_mp,InjCrv_tiPiI1Set_mp
  Compare To Constant : simulink/Logic and Bit Operations/Compare To Constant  relop=<=  const=0.02  OutDataTypeStr=boolean
  cmp_1 : RelationalOperator  Operator===  RndMeth=Nearest  InputSameDT=on
  cmp_3 : RelationalOperator  Operator===  RndMeth=Nearest  InputSameDT=on
  result_tws : ToWorkspace  VariableName=spec_result_002
  tws_1 : ToWorkspace  VariableName=spec_req_002_001
  tws_2 : ToWorkspace  VariableName=spec_req_002_002
  tws_3 : ToWorkspace  VariableName=spec_req_002_003
  result : Outport
  wires:
  sig_Req_Bus/1 -> BS_Req/1
  sig_Result_Bus/1 -> BS_Result/1
  AndN/1 -> result/1, result_tws/1
  BS_Req/1 -> cmp_1/1  "<testSig_InjCrv_qPiI1Set_mp>"
  BS_Result/1 -> cmp_1/2  "<InjCrv_qPiI1Set_mp>"
  cmp_1/1 -> tws_1/1, AndN/1
  BS_Req/2 -> Add/1  "<testSig_InjCrv_phiPiI1Set_mp>"
  BS_Result/2 -> Add/2  "<InjCrv_phiPiI1Set_mp>"
  Compare To Constant/1 -> tws_2/1, AndN/2
  BS_Req/3 -> cmp_3/1  "<testSig_InjCrv_tiPiI1Set_mp>"
  BS_Result/3 -> cmp_3/2  "<InjCrv_tiPiI1Set_mp>"
  cmp_3/1 -> tws_3/1, AndN/3
  Add/1 -> Compare To Constant/1

== system TST_InjCrv_PiIAddCor/compareSignals/Requirement_003/specifyOutputs ==
  sig_Req_Bus : Inport
  sig_Result_Bus : Inport  Port=2
  Add : Sum  Inputs=+-
  AndN : Logic  Inputs=3
  BS_Req : BusSelector  OutputSignals=testSig_InjCrv_qPiI1Set_mp,testSig_InjCrv_phiPiI1Set_mp,testSig_InjCrv_tiPiI1Set_mp
  BS_Result : BusSelector  OutputSignals=InjCrv_qPiI1Set_mp,InjCrv_phiPiI1Set_mp,InjCrv_tiPiI1Set_mp
  Compare To Constant : simulink/Logic and Bit Operations/Compare To Constant  relop=<=  const=0.02  OutDataTypeStr=boolean
  cmp_1 : RelationalOperator  Operator===  RndMeth=Nearest  InputSameDT=on
  cmp_3 : RelationalOperator  Operator===  RndMeth=Nearest  InputSameDT=on
  result_tws : ToWorkspace  VariableName=spec_result_003
  tws_1 : ToWorkspace  VariableName=spec_req_003_001
  tws_2 : ToWorkspace  VariableName=spec_req_003_002
  tws_3 : ToWorkspace  VariableName=spec_req_003_003
  result : Outport
  wires:
  sig_Req_Bus/1 -> BS_Req/1
  sig_Result_Bus/1 -> BS_Result/1
  AndN/1 -> result/1, result_tws/1
  BS_Req/1 -> cmp_1/1  "<testSig_InjCrv_qPiI1Set_mp>"
  BS_Result/1 -> cmp_1/2  "<InjCrv_qPiI1Set_mp>"
  cmp_1/1 -> tws_1/1, AndN/1
  BS_Req/2 -> Add/1  "<testSig_InjCrv_phiPiI1Set_mp>"
  BS_Result/2 -> Add/2  "<InjCrv_phiPiI1Set_mp>"
  Compare To Constant/1 -> tws_2/1, AndN/2
  BS_Req/3 -> cmp_3/1  "<testSig_InjCrv_tiPiI1Set_mp>"
  BS_Result/3 -> cmp_3/2  "<InjCrv_tiPiI1Set_mp>"
  cmp_3/1 -> tws_3/1, AndN/3
  Add/1 -> Compare To Constant/1
